simulink model "vRTHS_Referencia"  (R2021a)
settings: Solver=ode4  StartTime=0.0  StopTime=ttotal  FixedStep=dtsim  RelTol=1e-3
values from neighbouring files (symbols this model uses):
  Edificio = ss(ssA,[ssB1 ssB2],ssC,[ssD1 ssD2])    [vRTHS.m]
  params = parametros    [vRTHS.m]
  sys_kalman = sys_kalman(4:9,:)    [vRTHS.m]
  tipo_control = 3    [vRTHS.m]
undefined symbols (not defined in the file or in its folder): Kc
settings Model: Creator=cristobal  LastModifiedBy=maryf
settings SolverCC: AlgebraicLoopSolver=TrustRegion
settings DataIOCC: ReturnWorkspaceOutputs=off
settings DebuggingCC: SFMachineParentedDataDiag=warning  ArithmeticOperatorsInVariantConditions=warning
settings SFSimCC: SimUseLocalCustomCode=off  CustomCodeUndefinedFunction=UseInterfaceOnly
settings RTWCC: RTWUseLocalCustomCode=off
settings CodeAppCC: StateflowObjectComments=on

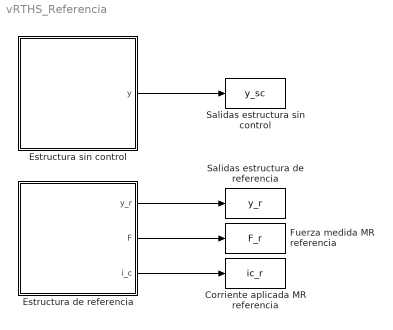
== system vRTHS_Referencia ==
  Corriente aplicada MR referencia : ToWorkspace  VariableName=ic_r  SaveFormat=Timeseries  SampleTime=-1
  Estructura de referencia : Subsystem
  Estructura sin control : Subsystem
  Fuerza medida MR referencia : ToWorkspace  VariableName=F_r  SaveFormat=Timeseries  SampleTime=-1
  Salidas estructura de referencia : ToWorkspace  VariableName=y_r  SaveFormat=Timeseries  SampleTime=-1
  Salidas estructura sin control : ToWorkspace  VariableName=y_sc  SaveFormat=Timeseries  SampleTime=-1
  wires:
  Estructura de referencia/1(y_r) -> Salidas estructura de referencia/1
  Estructura sin control/1(y) -> Salidas estructura sin control/1
  Estructura de referencia/2(F) -> Fuerza medida MR referencia/1
  Estructura de referencia/3(i_c) -> Corriente aplicada MR referencia/1

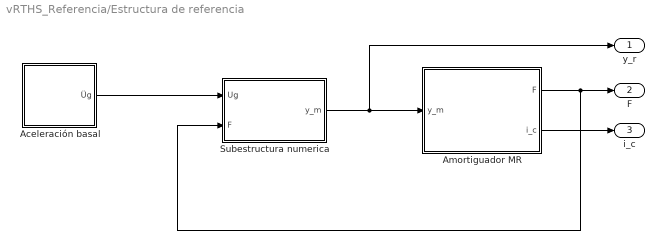
== system vRTHS_Referencia/Estructura de referencia ==
  Aceleración basal : Subsystem
  Amortiguador MR : Subsystem
  Subestructura numerica : Subsystem
  y_r : Outport  VectorParamsAs1DForOutWhenUnconnected=off
  F : Outport  Port=2  VectorParamsAs1DForOutWhenUnconnected=off
  i_c : Outport  Port=3  VectorParamsAs1DForOutWhenUnconnected=off
  wires:
  Amortiguador MR/1(F) -> Subestructura numerica/2("F "), F/1
  Subestructura numerica/1(y_m) -> y_r/1, Amortiguador MR/1(y_m)
  Amortiguador MR/2(i_c) -> i_c/1
  Aceleración basal/1(Üg) -> Subestructura numerica/1(Ug)

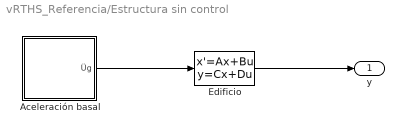
== system vRTHS_Referencia/Estructura sin control ==
  Aceleración basal : Subsystem
  Edificio : StateSpace  A=Edificio(:,1).A  B=Edificio(:,1).B  C=Edificio(:,1).C  D=Edificio(:,1).D  InitialCondition=0
  y : Outport  VectorParamsAs1DForOutWhenUnconnected=off
  wires:
  Edificio/1 -> y/1
  Aceleración basal/1(Üg) -> Edificio/1

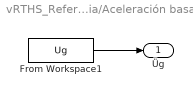
== system vRTHS_Referencia/Estructura de referencia/Aceleración basal ==
  From Workspace1 : FromWorkspace  VariableName=Ug  OutputAfterFinalValue=Setting to zero
  Üg : Outport  VectorParamsAs1DForOutWhenUnconnected=off
  wires:
  From Workspace1/1 -> Üg/1

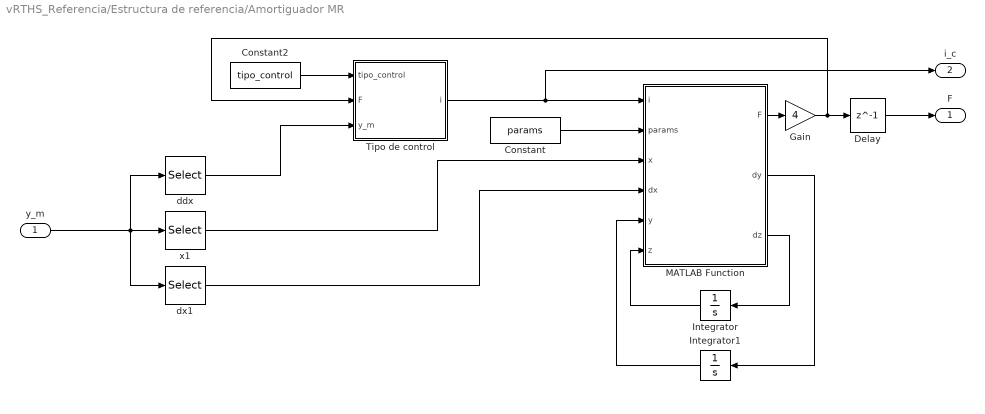
== system vRTHS_Referencia/Estructura de referencia/Amortiguador MR ==
  y_m : Inport
  Constant : Constant  Value=params
  Constant2 : Constant  Value=tipo_control
  Delay : Delay  DelayLength=1  InitialCondition=0
  Gain : Gain  Gain=4
  Integrator : Integrator
  Integrator1 : Integrator
  MATLAB Function : MATLAB Function  TreatAsAtomicUnit=on
  Tipo de control : Subsystem
  ddx : Selector  InputPortWidth=9  IndexOptions=Index vector (dialog)  Indices=7:9  OutputSizes=1
  dx1 : Selector  InputPortWidth=9  IndexOptions=Index vector (dialog)  Indices=4  OutputSizes=1
  x1 : Selector  InputPortWidth=9  IndexOptions=Index vector (dialog)  Indices=[1]  OutputSizes=1
  F : Outport
  i_c : Outport  Port=2
  wires:
  Tipo de control/1(i) -> i_c/1, MATLAB Function/1(i)
  Delay/1 -> F/1
  Gain/1 -> Tipo de control/2(F), Delay/1
  dx1/1 -> MATLAB Function/4(dx)
  ddx/1 -> Tipo de control/3(y_m)
  x1/1 -> MATLAB Function/3(x)
  MATLAB Function/1(F) -> Gain/1
  Integrator1/1 -> MATLAB Function/5(y)
  MATLAB Function/3(dz) -> Integrator/1
  Constant2/1 -> Tipo de control/1(tipo_control)
  Integrator/1 -> MATLAB Function/6(z)
  Constant/1 -> MATLAB Function/2(params)
  MATLAB Function/2(dy) -> Integrator1/1
  y_m/1 -> ddx/1, dx1/1, x1/1

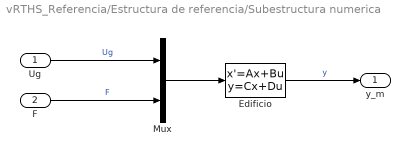
== system vRTHS_Referencia/Estructura de referencia/Subestructura numerica ==
  Ug : Inport
  "F " : Inport  Port=2
  Edificio : StateSpace  A=Edificio.A  B=Edificio.B  C=Edificio.C  D=Edificio.D  InitialCondition=0
  Mux : Mux  Inputs=2
  y_m : Outport
  wires:
  Edificio/1 -> y_m/1  "y"
  Mux/1 -> Edificio/1
  Ug/1 -> Mux/1  "Ug"
  "F "/1 -> Mux/2  "F"

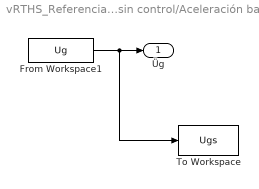
== system vRTHS_Referencia/Estructura sin control/Aceleración basal ==
  From Workspace1 : FromWorkspace  VariableName=Ug  OutputAfterFinalValue=Setting to zero
  To Workspace : ToWorkspace  VariableName=Ugs  SaveFormat=Timeseries  SampleTime=-1
  Üg : Outport  VectorParamsAs1DForOutWhenUnconnected=off
  wires:
  From Workspace1/1 -> To Workspace/1, Üg/1

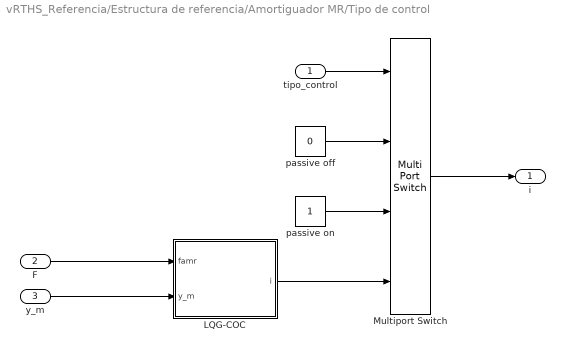
== system vRTHS_Referencia/Estructura de referencia/Amortiguador MR/Tipo de control ==
  tipo_control : Inport
  F : Inport  Port=2
  y_m : Inport  Port=3
  LQG-COC : Subsystem
  Multiport Switch : MultiPortSwitch
  passive off : Constant  Value=0
  passive on : Constant
  i : Outport
  wires:
  tipo_control/1 -> Multiport Switch/1
  Multiport Switch/1 -> i/1
  passive off/1 -> Multiport Switch/2
  passive on/1 -> Multiport Switch/3
  LQG-COC/1(i) -> Multiport Switch/4
  y_m/1 -> LQG-COC/2(y_m)
  F/1 -> LQG-COC/1(famr)

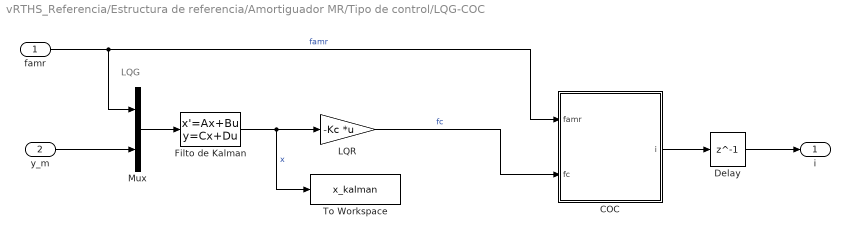
== system vRTHS_Referencia/Estructura de referencia/Amortiguador MR/Tipo de control/LQG-COC ==
  note: LQG
  famr : Inport
  y_m : Inport  Port=2
  COC : MATLAB Function  TreatAsAtomicUnit=on
  Delay : Delay  DelayLength=1  InitialCondition=0
  Filto de Kalman : StateSpace  A=sys_kalman.a  B=sys_kalman.b  C=sys_kalman.c  D=sys_kalman.d  InitialCondition=0
  LQR : Gain  Gain=-Kc  Multiplication=Matrix(K*u) (u vector)
  Mux : Mux  Inputs=2
  To Workspace : ToWorkspace  VariableName=x_kalman  SaveFormat=Timeseries  SampleTime=-1
  i : Outport
  wires:
  Mux/1 -> Filto de Kalman/1
  famr/1 -> COC/1(famr), Mux/1  "famr"
  y_m/1 -> Mux/2
  Filto de Kalman/1 -> To Workspace/1, LQR/1  "x"
  Delay/1 -> i/1
  COC/1(i) -> Delay/1
  LQR/1 -> COC/2(fc)  "fc"

== matlab function vRTHS_Referencia/Estructura de referencia/Amortiguador MR/Tipo de control/LQG-COC/COC ==
  data: famr input; i output; fc input
function i = fcn(famr,fc)
if abs(fc)>abs(famr)
    i = 1;
else
    i = 0;
end

== matlab function vRTHS_Referencia/Estructura de referencia/Amortiguador MR/MATLAB Function ==
  data: i input; params input; x input; dx input; y input; z input; F output size=1; dy output; dz output
function [F,dy,dz] = fcn(i,params,x,dx,y,z)
    A = 300;   
    n = 2;   
    k0 = params(1);
    k1 = params(2);
    x0 = params(3);
    alpha = params(4)*i^2+params(5)*i+params(6);
    gamma = params(7)*exp(params(8)*i);
    beta = gamma;
    c0 = params(9)*i+params(10);
    c1 = params(11)*i+params(12);

    x = x*1000; % el modelo está en mm N
    dx = dx*1000;
    dy = 1/(c0+c1)*(alpha*z+k0*(x-y)+c0*dx);
    dz = -gamma*abs(dx-dy)*((abs(z))^(n-1))*z-beta*(dx-dy)*(abs(z)^n)+A*(dx-dy);
    F  = c1*dy+k1*(x-x0);
